simulink model "oldFS_safetyTests"  (R2019a)
settings: Solver=FixedStepAuto  StartTime=0.0  StopTime=80  FixedStep=0.01  RelTol=1e-3
libraries: simulink x2, autolibshared x2, vehdynlibsteering x2, autolibutils x2, eeGeneralControl x1
settings Model: Creator=ckreienk  LastModifiedBy=ckreienk
settings DataIOCC: ReturnWorkspaceOutputs=off
settings DebuggingCC: ArithmeticOperatorsInVariantConditions=warning

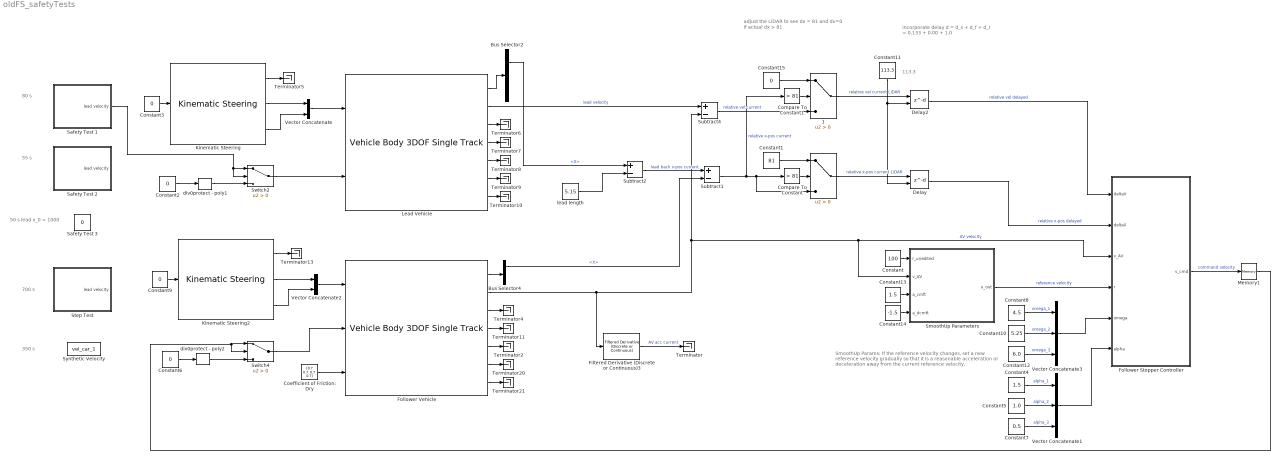
== system oldFS_safetyTests ==
  note: 113.3
  note: incorporate delay
      | d = d_s + d_f + d_r
      | = 0.133 + 0.00 + 1.0
  note: adjust the LiDAR to see
      | dx = 81 and dv=0
      | if actual dx > 81
  note: SmoothUp Params:
      | If the reference velocity changes,
      | set a new reference velocity gradually
      | so that it is a reasonable acceleration
      | or deceleration away from the current
      | reference velocity.
  note: 50 s
      | lead x_0 = 1000
  note: 80 s
  note: 700 s
  note: 350 s
  note: 55 s
  " " : Switch  Criteria=u2 > Threshold
  " 1" : Switch  Criteria=u2 > Threshold
  Bus Selector2 : BusSelector  OutputSignals=InertFrm.Geom.Disp.X,InertFrm.Geom.Disp.Y
  Bus Selector4 : BusSelector  OutputSignals=InertFrm.Geom.Disp.X,InertFrm.Geom.Disp.Y
  Coefficient of Friction: Dry : Constant  Value=[0.7 0.7; 0.7 0.7]
  Compare To Constant : simulink/Logic and Bit Operations/Compare To Constant  relop=>  const=81  OutDataTypeStr=boolean
  Compare To Constant1 : simulink/Logic and Bit Operations/Compare To Constant  relop=>  const=81  OutDataTypeStr=boolean
  Constant : Constant  Value=100
  Constant1 : Constant  Value=81
  Constant10 : Constant  Value=5.25
  Constant11 : Constant  Value=113.3
  Constant12 : Constant  Value=6.0
  Constant13 : Constant  Value=1.5
  Constant14 : Constant  Value=-1.5
  Constant{2..3,6,9,15} (5 alike) : Constant  Value=0
  Constant4 : Constant  Value=1.5
  Constant5 : Constant  Value=1.0
  Constant7 : Constant  Value=0.5
  Constant8 : Constant  Value=4.5
  Delay : Delay  DelayLengthSource=Input port  DelayLength=183
      settings: InputPortMap=u0,p1
  Delay2 : Delay  DelayLengthSource=Input port  DelayLength=183
      settings: InputPortMap=u0,p1
  Filtered Derivative (Discrete or Continuous)3 : eeGeneralControl/Filtered Derivative (Discrete or Continuous)  K=1  T=0.1  B=20  A=-20  minRatio=10  Ts=-1
      settings: SourceProductName=Simscape Electrical  SourceProductBaseCode=PS
  Follower Stopper Controller : Subsystem
  Follower Vehicle : autolibshared/Vehicle Body 3DOF Single Track  trackMode=Dual  inputMode=External longitudinal velocity  frontSteerMode=on  rearSteerMode=off  windMode=off  muMode=on  extFMode=off  extMMode=off  extXo=off  extpsio=off  extxdoto=off  extro=off  extYo=off  extTamb=off  extydoto=off  aMode=2  NF=2  NR=2  m=2000  a=1.4  b=1.6  h=0.35  X_o=0  xdot_o=0  CalphaMode=off  sigmaMode=on  d=0  w=[1.4,1.4]  Cy_f=12e3  Cy_r=11e3  sigma_f=.1  sigma_r=.1  alpha_f_brk=[-.1 .1]  Cy_f_data=[-9e3 9e3]  alpha_r_brk=[-.1 .1]  Cy_r_data=[-9e3 9e3]  Y_o=0  ydot_o=0  Izz=4000  psi_o=0  r_o=0  Af=2  Cd=.3  Cl=.1  Cpm=.1  beta_w=[0:0.01:0.3]  Cs=[0:0.03:0.9]  Cym=[0:0.01:0.3]  Pabs=101325  Tair=273  g=9.81  mu=1  xdot_tol=.01  Fznom=5000  Fxtire_sat=7e4  Fytire_sat=7e4  longOff=0  latOff=0  vertOff=0  wrapAng=off
      settings: SourceProductName=Powertrain Blockset  SourceProductBaseCode=PW
  Kinematic Steering : vehdynlibsteering/Kinematic Steering  StrgType=Ackerman  StrgRatioType=Constant  Loc=Front  NrmlFctr=0.01  TrckWdth=1  WhlBase=1.524  Db=0  StrgRng=1.25*pi  StrgAngBpts="[-6.2832   -5.0265   -3.7699   -2.5133   -1.2566         0    1.2566    2.5133    3.7699    5.0265    6.2832]"  StrgRatioTbl=|  StrgRatio=100  StrgArmLngth=0.1  RckCsLngth=0.5  TieRodLngth=0.248  D=0.2  PnnRadius=0.0057  PnnRadiusTbl="[0.0055    0.0055    0.0056    0.0057    0.0058    0.0057    0.0057    0.0057    0.0056    0.0055    0.0055]"  RodLngth=0.1  ParaArmLngth=0.9  aMode=2
      | [13.5000   13.3750   13.2500   13.1250   13.0000   13.0000   13.0000   13.1250   13.2500   13.3750   13.5000
      | ]
      settings: SourceProductName=Vehicle Dynamics Blockset
  Kinematic Steering2 : vehdynlibsteering/Kinematic Steering  StrgType=Ackerman  StrgRatioType=Constant  Loc=Front  NrmlFctr=0.01  TrckWdth=1  WhlBase=1.524  Db=0  StrgRng=1.25*pi  StrgAngBpts="[-6.2832   -5.0265   -3.7699   -2.5133   -1.2566         0    1.2566    2.5133    3.7699    5.0265    6.2832]"  StrgRatioTbl=|  StrgRatio=100  StrgArmLngth=0.1  RckCsLngth=0.5  TieRodLngth=0.248  D=0.2  PnnRadius=0.0057  PnnRadiusTbl="[0.0055    0.0055    0.0056    0.0057    0.0058    0.0057    0.0057    0.0057    0.0056    0.0055    0.0055]"  RodLngth=0.1  ParaArmLngth=0.9  aMode=2
      | [13.5000   13.3750   13.2500   13.1250   13.0000   13.0000   13.0000   13.1250   13.2500   13.3750   13.5000
      | ]
      settings: SourceProductName=Vehicle Dynamics Blockset
  Lead Vehicle : autolibshared/Vehicle Body 3DOF Single Track  trackMode=Dual  inputMode=External longitudinal velocity  frontSteerMode=on  rearSteerMode=off  windMode=off  muMode=off  extFMode=off  extMMode=off  extXo=off  extpsio=off  extxdoto=off  extro=off  extYo=off  extTamb=off  extydoto=off  aMode=2  NF=2  NR=2  m=2000  a=1.4  b=1.6  h=0.35  X_o=10  xdot_o=0  CalphaMode=off  sigmaMode=on  d=0  w=[1.4,1.4]  Cy_f=12e3  Cy_r=11e3  sigma_f=.1  sigma_r=.1  alpha_f_brk=[-.1 .1]  Cy_f_data=[-9e3 9e3]  alpha_r_brk=[-.1 .1]  Cy_r_data=[-9e3 9e3]  Y_o=0  ydot_o=0  Izz=4000  psi_o=0  r_o=0  Af=2  Cd=.3  Cl=.1  Cpm=.1  beta_w=[0:0.01:0.3]  Cs=[0:0.03:0.9]  Cym=[0:0.01:0.3]  Pabs=101325  Tair=273  g=9.81  mu=1  xdot_tol=.01  Fznom=5000  Fxtire_sat=7e4  Fytire_sat=7e4  longOff=0  latOff=0  vertOff=0  wrapAng=off
      settings: SourceProductName=Powertrain Blockset  SourceProductBaseCode=PW
  Memory1 : Memory
  Safety Test 1 : Subsystem
  Safety Test 2 : Subsystem
  Safety Test 3 : Constant  Value=0
  SmoothUp Parameters : MATLAB Function  TreatAsAtomicUnit=on
  Step Test : Subsystem
  Subtract1 : Sum  Inputs=+-
  Subtract2 : Sum  Inputs=+-
  Subtract4 : Sum  Inputs=+-
  Switch2 : Switch  Criteria=u2 > Threshold
  Switch4 : Switch  Criteria=u2 > Threshold
  Synthetic Velocity : FromWorkspace  VariableName=vel_car_1
  Terminator{,2,4..11,13,20..21} (13 alike) : Terminator
  Vector Concatenate : Concatenate
  Vector Concatenate1 : Concatenate  NumInputs=3
  Vector Concatenate2 : Concatenate
  Vector Concatenate3 : Concatenate  NumInputs=3
  div0protect - poly1 : autolibutils/div0protect - poly  thresh=1e-3  aMode=2
      settings: SourceProductName=Powertrain Blockset  SourceProductBaseCode=PW
  div0protect - poly2 : autolibutils/div0protect - poly  thresh=1e-3  aMode=2
      settings: SourceProductName=Powertrain Blockset  SourceProductBaseCode=PW
  lead length : Constant  Value=5.15
  wires:
  Vector Concatenate/1 -> Lead Vehicle/1
  Lead Vehicle/7 -> Terminator10/1
  Lead Vehicle/6 -> Terminator9/1
  Lead Vehicle/5 -> Terminator8/1
  Lead Vehicle/4 -> Terminator7/1
  Lead Vehicle/3 -> Terminator6/1
  Kinematic Steering/3 -> Vector Concatenate/2
  Kinematic Steering/2 -> Vector Concatenate/1
  Kinematic Steering/1 -> Terminator5/1
  Constant3/1 -> Kinematic Steering/1
  Switch2/1 -> Lead Vehicle/2
  div0protect - poly1/1 -> Switch2/3
  Constant2/1 -> div0protect - poly1/1
  Lead Vehicle/1 -> Bus Selector2/1
  Compare To Constant/1 -> " "/2
  Follower Stopper Controller/1(v_cmd) -> Memory1/1  "command velocity"
  Vector Concatenate2/1 -> Follower Vehicle/1
  Delay2/1 -> Follower Stopper Controller/1(deltaV)  "relative vel delayed"
  Memory1/1 -> Switch4/2, Switch4/1
  Coefficient of Friction: Dry/1 -> Follower Vehicle/3
  Delay/1 -> Follower Stopper Controller/2(deltaX)  "relative x-pos delayed"
  Follower Vehicle/4 -> Terminator11/1
  Bus Selector2/1 -> Subtract2/1  "<X>"
  Kinematic Steering2/3 -> Vector Concatenate2/2
  Switch4/1 -> Follower Vehicle/2
  " "/1 -> Delay/1  "relative x-pos current LiDAR"
  Follower Vehicle/1 -> Bus Selector4/1
  Constant1/1 -> " "/1
  Constant/1 -> SmoothUp Parameters/1(r_unedited)
  Lead Vehicle/2 -> Subtract4/1  "lead velocity"
  Kinematic Steering2/1 -> Terminator13/1
  Follower Vehicle/7 -> Terminator21/1
  SmoothUp Parameters/1(u_out) -> Follower Stopper Controller/4(r)  "reference velocity"
  Kinematic Steering2/2 -> Vector Concatenate2/1
  Follower Vehicle/3 -> Terminator4/1
  Follower Vehicle/6 -> Terminator20/1
  Constant9/1 -> Kinematic Steering2/1
  Constant6/1 -> div0protect - poly2/1
  lead length/1 -> Subtract2/2
  Subtract2/1 -> Subtract1/1  "lead back x-pos current"
  Follower Vehicle/2 -> Filtered Derivative (Discrete or Continuous)3/1, SmoothUp Parameters/2(v_AV), Follower Stopper Controller/3(v_AV), Subtract4/2  "AV velocity"
  Constant11/1 -> Delay/2, Delay2/2
  Bus Selector4/1 -> Subtract1/2  "<X>"
  div0protect - poly2/1 -> Switch4/3
  Follower Vehicle/5 -> Terminator2/1
  Constant4/1 -> Vector Concatenate1/1  "alpha_1"
  Constant5/1 -> Vector Concatenate1/2  "alpha_2"
  Vector Concatenate1/1 -> Follower Stopper Controller/6(alpha)
  Constant7/1 -> Vector Concatenate1/3  "alpha_3"
  Constant10/1 -> Vector Concatenate3/2  "omega_2"
  Vector Concatenate3/1 -> Follower Stopper Controller/5(omega)
  Constant12/1 -> Vector Concatenate3/3  "omega_3"
  Constant8/1 -> Vector Concatenate3/1  "omega_1"
  Constant13/1 -> SmoothUp Parameters/3(a_cmft)
  Constant14/1 -> SmoothUp Parameters/4(a_dcmft)
  Subtract4/1 -> " 1"/3  "relative vel current"
  Constant15/1 -> " 1"/1
  Compare To Constant1/1 -> " 1"/2
  " 1"/1 -> Delay2/1  "relative vel current LiDAR"
  Subtract1/1 -> " "/3, Compare To Constant/1, Compare To Constant1/1  "relative x-pos current"
  Filtered Derivative (Discrete or Continuous)3/1 -> Terminator/1  "AV acc current"
  Safety Test 1/1(lead velocity) -> Switch2/1, Switch2/2

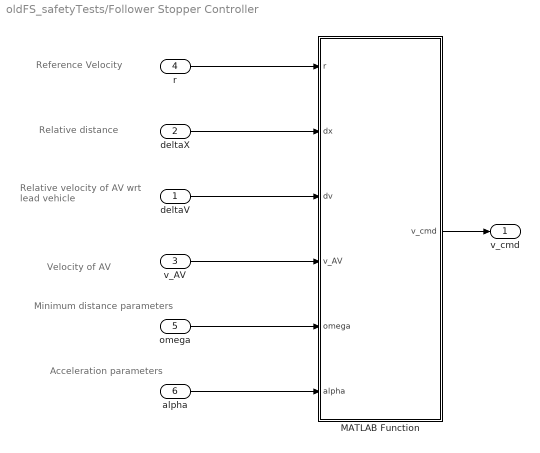
== system oldFS_safetyTests/Follower Stopper Controller ==
  note: Relative distance
  note: Reference Velocity
  note: Velocity of AV
  note: Relative velocity of
      | AV wrt lead vehicle
  note: Minimum distance
      | parameters
  note: Acceleration
      | parameters
  deltaV : Inport
  deltaX : Inport  Port=2
  v_AV : Inport  Port=3
  r : Inport  Port=4
  omega : Inport  Port=5
  alpha : Inport  Port=6
  MATLAB Function : MATLAB Function  TreatAsAtomicUnit=on
  v_cmd : Outport
  wires:
  r/1 -> MATLAB Function/1(r)
  v_AV/1 -> MATLAB Function/4(v_AV)
  MATLAB Function/1(v_cmd) -> v_cmd/1
  deltaV/1 -> MATLAB Function/3(dv)
  deltaX/1 -> MATLAB Function/2(dx)
  omega/1 -> MATLAB Function/5(omega)
  alpha/1 -> MATLAB Function/6(alpha)

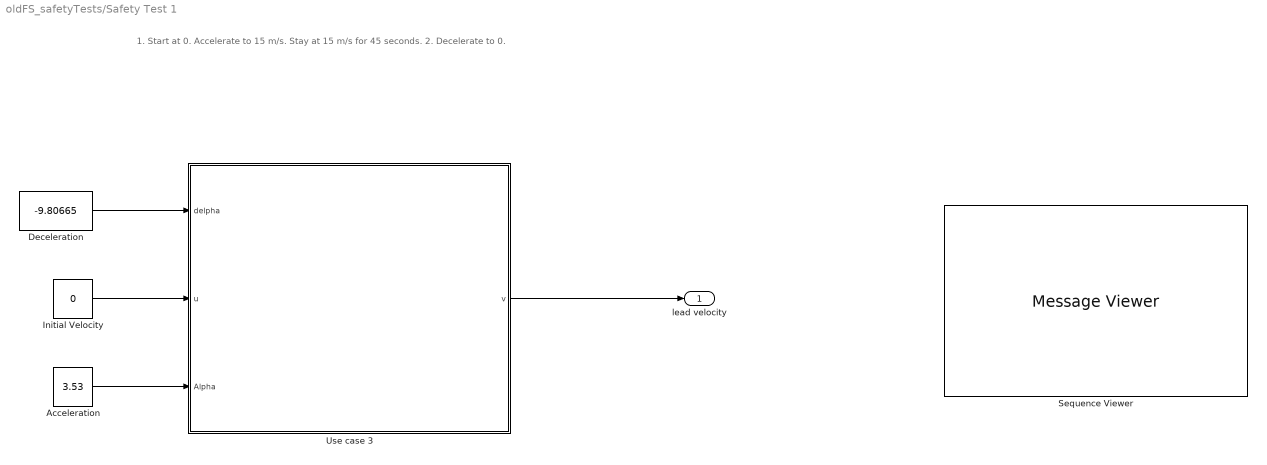
== system oldFS_safetyTests/Safety Test 1 ==
  note: 1. Start at 0. Accelerate to 15 m/s. Stay at 15 m/s for 45 seconds.
      | 2. Decelerate to 0.
  Acceleration : Constant  Value=3.53
  Deceleration : Constant  Value=-9.80665
  Initial Velocity : Constant  Value=0
  Sequence Viewer : MessageViewer
  Use case 3 : Stateflow chart  TreatAsAtomicUnit=on
  lead velocity : Outport
  wires:
  Acceleration/1 -> Use case 3/3(Alpha)
  Initial Velocity/1 -> Use case 3/2(u)
  Deceleration/1 -> Use case 3/1(delpha)
  Use case 3/1(v) -> lead velocity/1

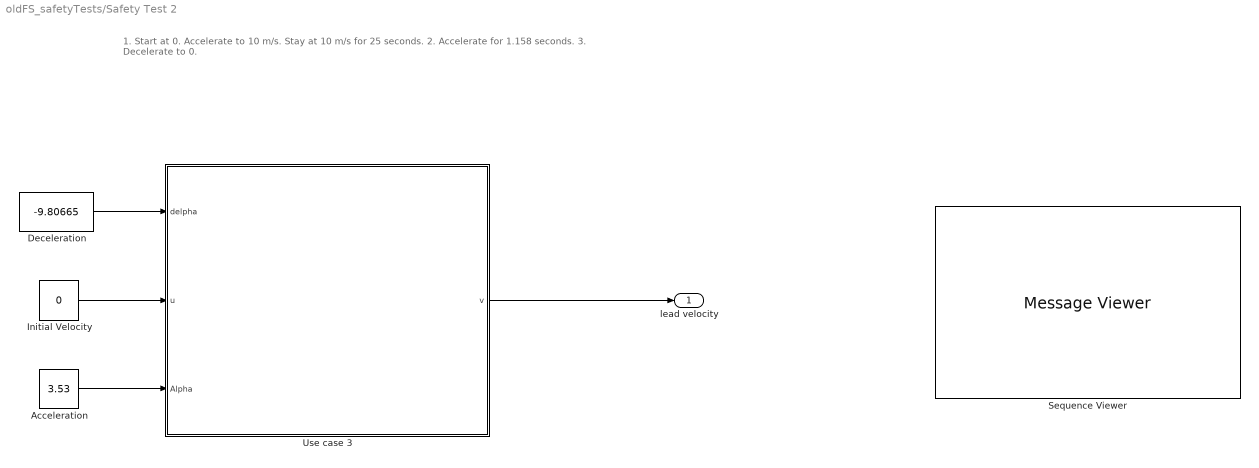
== system oldFS_safetyTests/Safety Test 2 ==
  note: 1. Start at 0. Accelerate to 10 m/s. Stay at 10 m/s for 25 seconds.
      | 2. Accelerate for 1.158 seconds.
      | 3. Decelerate to 0.
  Acceleration : Constant  Value=3.53
  Deceleration : Constant  Value=-9.80665
  Initial Velocity : Constant  Value=0
  Sequence Viewer : MessageViewer
  Use case 3 : Stateflow chart  TreatAsAtomicUnit=on
  lead velocity : Outport
  wires:
  Use case 3/1(v) -> lead velocity/1
  Deceleration/1 -> Use case 3/1(delpha)
  Initial Velocity/1 -> Use case 3/2(u)
  Acceleration/1 -> Use case 3/3(Alpha)

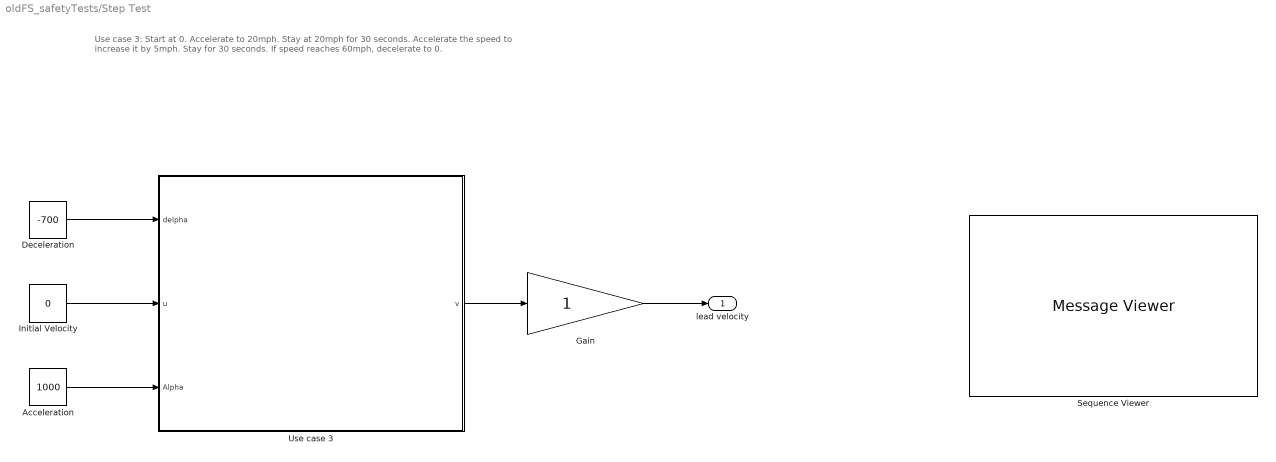
== system oldFS_safetyTests/Step Test ==
  note: Use case 3:
      | Start at 0. Accelerate to 20mph. Stay at 20mph for 30 seconds.
      | Accelerate the speed to increase it by 5mph. Stay for 30 seconds.
      | If speed reaches 60mph, decelerate to 0.
  Acceleration : Constant  Value=1000
  Deceleration : Constant  Value=-700
  Gain : Gain
  Initial Velocity : Constant  Value=0
  Sequence Viewer : MessageViewer
  Use case 3 : Stateflow chart  TreatAsAtomicUnit=on
  lead velocity : Outport
  wires:
  Use case 3/1(v) -> Gain/1
  Acceleration/1 -> Use case 3/3(Alpha)
  Initial Velocity/1 -> Use case 3/2(u)
  Deceleration/1 -> Use case 3/1(delpha)
  Gain/1 -> lead velocity/1

== stateflow chart oldFS_safetyTests/Safety Test 2/Use case 3 ==
  state Hold
    entry: u2 = v;
    during: v = u2;
    exit:
    note: HOLD STATE
  state Accelerate
    entry: entryState = 1; v = 0;
    during: v = getNewVaccel(v, Alpha)
    exit:  nextState = entryState + 1;
    note: STATE 1
  state Accelerate1
    entry: entryState = nextState; v = u2;
    during: v = getNewVaccel(v, Alpha);
    exit: nextState = entryState + 1;
    note: STATE 2
  state Decelerate
    entry: entryState = nextState; v = u2;
    during: v = getNewVdecel(v,delpha);
    exit: nextState = entryState + 1;
    note: STATE 3
  state Hold1
    entry:
    during: v = 0;
    exit:
  state zero
    entry: v = 0;
    during:v = 0;
    note: STATE 4
  (default) -> Accelerate
  Hold -> Accelerate1 : [after(25, sec)]
  Accelerate -> Hold : [v>=10 ]
  Accelerate1 -> Decelerate : [after(1.158, sec)]
  Decelerate -> Hold1 : [v==0]
  Hold1 -> zero
  data: init_velocity function_input; deceleration function_input; new_vel function_output; init_velocity function_input; acceleration function_input; new_vel function_output; delpha input; u input; Alpha input; v output =0; u2 local =0; entryState local =0; nextState local =0
  function new_vel = getNewVdecel(init_velocity, deceleration):
    | function new_vel = getNewVdecel(init_velocity, deceleration)
    | 
    | new_vel = init_velocity - abs(deceleration*0.01);
    | new_vel = max(new_vel,0);
    | 
    | end
  function new_vel = getNewVaccel(init_velocity, acceleration):
    | function new_vel = getNewVaccel(init_velocity, acceleration)
    | 
    | new_vel = init_velocity + (acceleration*0.01);
    | 
    | end

== stateflow chart oldFS_safetyTests/Safety Test 1/Use case 3 ==
  state zero
    entry: v = 0;
    during:v = 0;
    note: STATE 4
  state Hold
    entry: u2 = v;
    during: v = u2;
    exit:
    note: HOLD STATE
  state AccelerateTo60_init
    entry: entryState = 1; v = 0;
    during: v = getNewVaccel(v, Alpha)
    exit:  nextState = entryState + 1;
    note: STATE 1
  state Hold1
    entry:
    during: v = 0;
    exit:
  state Accelerate
    entry: entryState = nextState; v = u2;
    during: v = getNewVdecel(v,delpha);
    exit: nextState = entryState + 1;
    note: STATE 2
  Hold1 -> zero
  (default) -> AccelerateTo60_init
  Hold -> Accelerate : [after(45, sec)]
  AccelerateTo60_init -> Hold : [v>=15 ]
  Accelerate -> Hold1 : [v==0]
  data: init_velocity function_input; deceleration function_input; new_vel function_output; init_velocity function_input; acceleration function_input; new_vel function_output; delpha input; u input; Alpha input; v output =0; u2 local =0; entryState local =0; nextState local =0
  function new_vel = getNewVdecel(init_velocity, deceleration):
    | function new_vel = getNewVdecel(init_velocity, deceleration)
    | 
    | new_vel = init_velocity - abs(deceleration*0.01);
    | new_vel = max(new_vel,0);
    | 
    | end
  function new_vel = getNewVaccel(init_velocity, acceleration):
    | function new_vel = getNewVaccel(init_velocity, acceleration)
    | 
    | new_vel = init_velocity + (acceleration*0.01);
    | 
    | end

== matlab function oldFS_safetyTests/Follower Stopper Controller/MATLAB Function ==
  settings: updateMethod=DISCRETE
  data: r input; v_cmd output; dx input; dv input; v_AV input; omega input; alpha input
function v_cmd = fcn(r,dx,dv,v_AV,...
    omega,alpha)
%#codegen
% Safety controller, based on quadratic bands.
% Input: r = desired velocity (from other models)
%          dx = estimate of gap to vehicle ahead
%          dv = estimate of time derivative of dx (= velocity difference)
%         v_AV = velocity of AV
%      dx_min = minimum distance
% dx_activate = distance below which controller does something
%       decel = vector of three deceleration values for parabolas
% Out:  u_cmd = actual velocity commanded (always u_cmd<=U)
%

% Lead vehicle velocity
v_lead = v_AV+dv; % velocity of lead vehicle
v_lead = max(v_lead,0); % lead vehicle cannot go backwards
v = min(r,v_lead); % safety velocity cannot exceed desired velocity U

% Treatment of positive dv-values
dv = min(dv,0); % domains for dv>0 same as dv=0

% For given dv, dx-values of band boundaries
dx1 = omega(1)+1/(2*alpha(1))*dv.^2;
dx2 = omega(2)+1/(2*alpha(2))*dv.^2;
dx3 = omega(3)+1/(2*alpha(3))*dv.^2;

% Actual commanded velocity
new_cmd = double((dx<=dx1).*(0))+...
    (dx1<dx&dx<=dx2).*(v*(dx-dx1)/(dx2-dx1))+...
    (dx2<dx&dx<=dx3).*(v + (r-v)*(dx-dx2)/(dx3-dx2))+...
    (dx3<dx).*(r);

% Edit new_cmd to be a reasonable value based on the maximum acceleration
% and deceleration of the Ford Escape Hybrid
dt = 0.01;
possibleAcc = v_AV + 3.53*dt;
possibleDec = v_AV - 7.66*dt;
v_cmd = min(max(new_cmd, possibleDec), possibleAcc);

== matlab function oldFS_safetyTests/SmoothUp Parameters ==
  settings: updateMethod=DISCRETE
  data: r_unedited input; u_out output; v_AV input; a_cmft input; a_dcmft input
function u_out = fcn(r_unedited,v_AV,a_cmft,a_dcmft)
% #codegen
persistent y

if isempty(y)
    y=v_AV;
end

dt=0.01;
if( y > r_unedited + a_cmft*dt)
    y = max(r_unedited,y - abs(a_dcmft)*dt);
elseif( y < r_unedited - abs(a_dcmft)*dt)
    y = min(r_unedited,y + a_cmft*dt);
else
    y = r_unedited;
end

u_out = y;

== stateflow chart oldFS_safetyTests/Step Test/Use case 3 ==
  note: Use case 3:
      | Start at 0. Accelerate to 20mph. Stay at 20mph for 30 seconds.
      | Accelerate the speed to increase it by 5mph. Stay for 30 seconds.
      | If speed reaches 60mph, decelerate to 0.
  state zero
    entry: v = 0;
    during:v = 0;
    note: STATE 4
  state Hold
    entry: u2 = v;
    during: v = u2;
    exit:
    note: HOLD STATE
  state AccelerateTo60_init
    entry: entryState = 1; v = 0;
    during: v = getNewVaccel(v, Alpha)
    exit:  nextState = entryState + 1;
    note: STATE 1
  state Hold1
    entry:
    during: v = 3;
    exit:
  state Accelerate
    entry: entryState = nextState; v = u2;
    during: v = getNewVdecel(v,delpha);
    exit: nextState = entryState + 1;
    note: STATE 2
  note: 30 mph
  state Hold2
    entry: u2 = v;
    during: v = u2;
    exit:
    note: HOLD STATE
  note: 45 mph
  state AccelerateTo60_init1
    entry: entryState = 1; v = 3;
    during: v = getNewVaccel(v, Alpha)
    exit:  nextState = entryState + 1;
    note: STATE 1
  state Accelerate1
    entry: entryState = nextState; v = u2;
    during: v = getNewVdecel(v,delpha);
    exit: nextState = entryState + 1;
    note: STATE 2
  state Hold3
    entry:
    during: v = 0;
    exit:
  Hold3 -> zero : [v==0]
  (default) -> AccelerateTo60_init
  Hold -> Accelerate : [after(350, sec)]
  AccelerateTo60_init -> Hold : [v>=10]
  Accelerate -> Hold1 : [v==3]
  Hold1 -> AccelerateTo60_init1 : [after(150, sec)]
  Hold2 -> Accelerate1 : [after(600, sec)]
  AccelerateTo60_init1 -> Hold2 : [v>=20 ]
  Accelerate1 -> Hold3 : [v==0]
  data: init_velocity function_input; deceleration function_input; new_vel function_output; init_velocity function_input; acceleration function_input; new_vel function_output; delpha input; u input; Alpha input; v output =0; u2 local =0; entryState local =0; nextState local =0
  function new_vel = getNewVdecel(init_velocity, deceleration):
    | function new_vel = getNewVdecel(init_velocity, deceleration)
    | 
    | new_vel = init_velocity - abs(deceleration*0.01);
    | new_vel = max(new_vel,0);
    | 
    | end
  function new_vel = getNewVaccel(init_velocity, acceleration):
    | function new_vel = getNewVaccel(init_velocity, acceleration)
    | 
    | new_vel = init_velocity + (acceleration*0.01);
    | 
    | end
